simulink model "commu2"  (R2022a)
settings: Solver=FixedStepAuto  StartTime=0.0  StopTime=inf  RelTol=1e-3
libraries: instrumentseriallib x4, slrealtimeseriallib x2, hdlsllib x2, simulink x2
settings Model: Creator=imark  LastModifiedBy=weera
settings DebuggingCC: UnconnectedInputMsg=warning  UnconnectedOutputMsg=warning  UnconnectedLineMsg=warning
settings RTWCC: DLArmComputeVersion=19.05

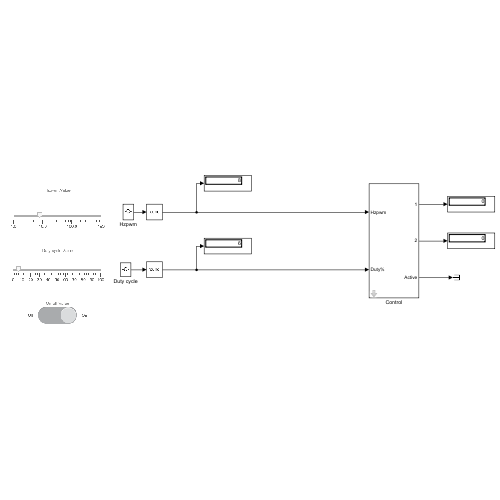
[thumbnail: Simulink's stored preview of the top-level diagram]
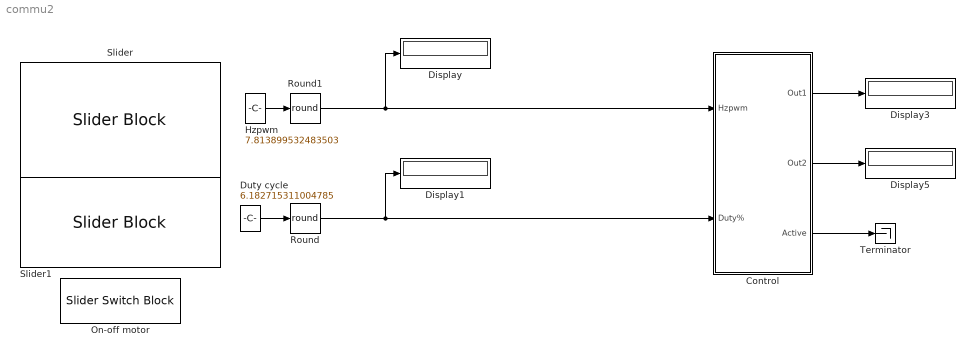
== system commu2 ==
  Control : Subsystem  mask{hz=1}
      mask prompts: hz "Sample rate"
  Display{,1,3,5} (4 alike) : Display
  Duty cycle : Constant  Value=6.182715311004785
  Hzpwm : Constant  Value=7.813899532483503
  On-off motor : SliderSwitchBlock
      settings: Values={{'Off', 'On'}, [0 1]}
  Round : Rounding  Operator=round
  Round1 : Rounding  Operator=round
  Slider : SliderBlock  ScaleMin=1  ScaleMax=1000  ScaleType=Log
  Slider1 : SliderBlock  TickInterval=10
  Terminator : Terminator
  wires:
  Duty cycle/1 -> Round/1
  Round/1 -> Display1/1, Control/2(Duty%)
  Hzpwm/1 -> Round1/1
  Round1/1 -> Display/1, Control/1(Hzpwm)
  Control/1(Out1) -> Display3/1
  Control/2(Out2) -> Display5/1
  Control/3(Active) -> Terminator/1

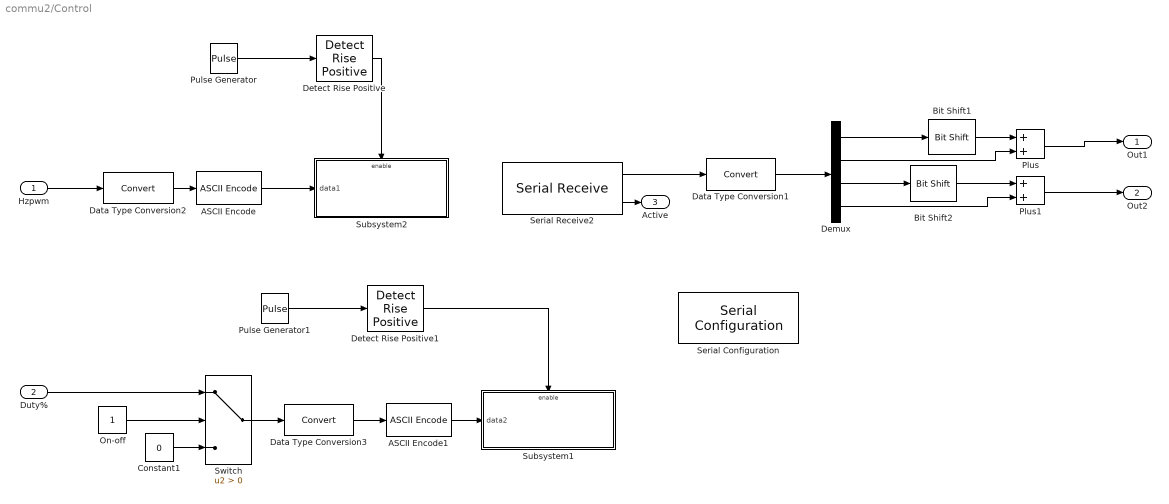
== system commu2/Control ==
  Hzpwm : Inport
  Duty% : Inport  Port=2
  ASCII Encode : slrealtimeseriallib/ASCII Encode  format=%c  nvars=1  maxlength=2  vartypes={ 'double' }
      settings: SourceProductBaseCode=XP
  ASCII Encode1 : slrealtimeseriallib/ASCII Encode  format=%c  nvars=1  maxlength=2  vartypes={ 'double' }
      settings: SourceProductBaseCode=XP
  Bit Shift1 : hdlsllib/Logic and Bit Operations/Bit Shift  mode=Shift Left Logical  N=8
  Bit Shift2 : hdlsllib/Logic and Bit Operations/Bit Shift  mode=Shift Left Logical  N=8
  Constant1 : Constant  Value=0
  Data Type Conversion1 : DataTypeConversion  SaturateOnIntegerOverflow=off  RndMeth=Floor
  Data Type Conversion2 : DataTypeConversion  SaturateOnIntegerOverflow=off  RndMeth=Floor
  Data Type Conversion3 : DataTypeConversion  SaturateOnIntegerOverflow=off  RndMeth=Floor
  Demux : Demux
  Detect Rise Positive : simulink/Logic and Bit Operations/Detect Rise Positive  vinit=0  OutDataTypeStr=boolean
  Detect Rise Positive1 : simulink/Logic and Bit Operations/Detect Rise Positive  vinit=0  OutDataTypeStr=boolean
  On-off : Constant
  Plus : Sum
  Plus1 : Sum
  Pulse Generator : DiscretePulseGenerator  PulseType=Time based  Period=1/hz  PulseWidth=50
  Pulse Generator1 : DiscretePulseGenerator  PulseType=Time based  Period=1/hz  PulseWidth=50  PhaseDelay=1/(hz*2)
  Serial Configuration : instrumentseriallib/Serial Configuration  Priority=-200000  PortSel=COM1  Port=COM1  ComPort=COM1  BaudRate=115200  DataBits=8  Parity=none  StopBits=1  ByteOrder=little-endian  FlowControl=none  Timeout=10  SimulateUsing=Interpreted execution  BlockInModel=on  aMode=1
      settings: SourceProductBaseCode=OT,IC,MT
  Serial Receive2 : instrumentseriallib/Serial Receive  Priority=1  PortSel=COM1  Port=COM1  ComPort=COM1  DataType=uint8  SaveDataType=uint8  ToggleHeader=on  Header=[73 109 64 99]  ToggleTerminator=on  Terminator=Custom terminator  CustomTerminator=[126]  InputFormat=Column major  ToggleDataSize=on  DataSize=[4]  EnableBlockingMode=off  ActionDataUnavailable=Output last received value  ActionWhenDataUnavailable=Output last received value  CustomValue=0  SampleTime=1/100  SimulateUsing=Interpreted execution  BlockInModel=on  aMode=1
      settings: SourceProductBaseCode=OT,IC,MT
  Subsystem1 : Subsystem
  Subsystem2 : Subsystem
  Switch : Switch  Criteria=u2 > Threshold  SaturateOnIntegerOverflow=off  InputSameDT=off
  Out1 : Outport
  Out2 : Outport  Port=2
  Active : Outport  Port=3
  wires:
  Plus1/1 -> Out2/1
  Plus/1 -> Out1/1
  Bit Shift2/1 -> Plus1/1
  Demux/3 -> Bit Shift2/1
  Data Type Conversion1/1 -> Demux/1
  Serial Receive2/2 -> Active/1
  Serial Receive2/1 -> Data Type Conversion1/1
  Bit Shift1/1 -> Plus/1
  Demux/4 -> Plus1/2
  Demux/2 -> Plus/2
  Demux/1 -> Bit Shift1/1
  On-off/1 -> Switch/2
  Data Type Conversion3/1 -> ASCII Encode1/1
  ASCII Encode/1 -> Subsystem2/1(data1)
  Duty%/1 -> Switch/1
  Detect Rise Positive1/1 -> Subsystem1/Enable
  ASCII Encode1/1 -> Subsystem1/1(data2)
  Switch/1 -> Data Type Conversion3/1
  Constant1/1 -> Switch/3
  Hzpwm/1 -> Data Type Conversion2/1
  Data Type Conversion2/1 -> ASCII Encode/1
  Pulse Generator/1 -> Detect Rise Positive/1
  Detect Rise Positive/1 -> Subsystem2/Enable
  Pulse Generator1/1 -> Detect Rise Positive1/1

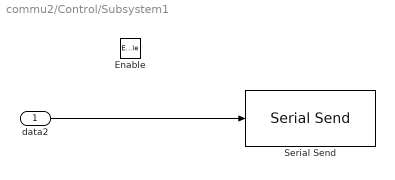
== system commu2/Control/Subsystem1 ==
  data2 : Inport
  Enable : EnablePort
  Serial Send : instrumentseriallib/Serial Send  Priority=1  PortSel=COM1  Port=COM1  ComPort=COM1  Header=[4 15]  Terminator=<none>  CustomTerminator=[127]  EnableBlockingMode=on  SimulateUsing=Interpreted execution  BlockInModel=on  aMode=1
      settings: SourceProductBaseCode=OT,IC,MT
  wires:
  data2/1 -> Serial Send/1

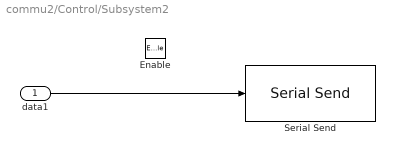
== system commu2/Control/Subsystem2 ==
  data1 : Inport
  Enable : EnablePort
  Serial Send : instrumentseriallib/Serial Send  Priority=1  PortSel=COM1  Port=COM1  ComPort=COM1  Header=[2 13]  Terminator=<none>  CustomTerminator=[126]  EnableBlockingMode=on  SimulateUsing=Interpreted execution  BlockInModel=on  aMode=1
      settings: SourceProductBaseCode=OT,IC,MT
  wires:
  data1/1 -> Serial Send/1
